simulink library "lib_Convection_LamFlatPlate"  (R2015a)
settings: Solver=ode45  StartTime=0.0  StopTime=10.0  RelTol=1e-3
libraries: simulink x1
settings Model: Creator=jlkratz  LastModifiedBy=jlkratz

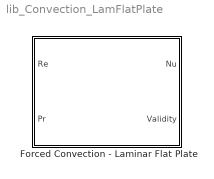
== system lib_Convection_LamFlatPlate ==
  Forced Convection - Laminar Flat Plate : Subsystem  mask(TSAT: Forced Convection - Laminar Flat Plate){LocalOrAvg_M=Average Nusselt number, IsothermOrIsoflux_M=Isothermal Plate}
      mask help:
      | This block estimates the Nusselt number of a laminar external flow over an isothermal or isoflux flat plate. It can either calculate the local or average Nusselt number over 1 surface of the plate. If the average Nusselt number is to be calcualted then assure the charateristic length used to calculate the Reynolds Number is the full length of the plate. Note that all fluid properrties should be evaluated at film temperature (average of the bulk fluid and surface temperatures). Beyond the flow being laminar the implemented correlations also requires:
      |
      | Pr >= 0.6
      |
      | If this contraint is not met then the "Validity" output will be 1, and otherwise will be 0. For more information on the implemented correlations and function of the block, see the block help menu.
      mask Help: web(which('Convection_TSAT_LaminarFlatPlate.html'),'-helpbrowser')
      mask TypeOptions LocalOrAvg_M: Local Nusselt number | Average Nusselt number
      mask TypeOptions IsothermOrIsoflux_M: Isothermal Plate | Isoflux Plate

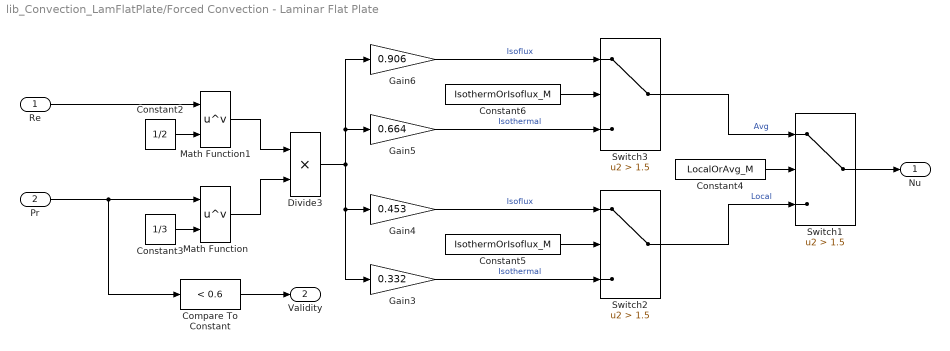
== system lib_Convection_LamFlatPlate/Forced Convection - Laminar Flat Plate ==
  Re : Inport
  Pr : Inport  Port=2
  Compare To Constant : simulink/Logic and Bit Operations/Compare To Constant  relop=<  const=0.6  OutDataTypeStr=boolean
  Constant2 : Constant  Value=1/2
  Constant3 : Constant  Value=1/3
  Constant4 : Constant  Value=LocalOrAvg_M
  Constant5 : Constant  Value=IsothermOrIsoflux_M
  Constant6 : Constant  Value=IsothermOrIsoflux_M
  Divide3 : Product  Inputs=**
  Gain3 : Gain  Gain=0.332
  Gain4 : Gain  Gain=0.453
  Gain5 : Gain  Gain=0.664
  Gain6 : Gain  Gain=0.906
  Math Function : Math  Operator=pow  SaturateOnIntegerOverflow=on
  Math Function1 : Math  Operator=pow  SaturateOnIntegerOverflow=on
  Switch1 : Switch  Criteria=u2 > Threshold  Threshold=1.5
  Switch2 : Switch  Criteria=u2 > Threshold  Threshold=1.5
  Switch3 : Switch  Criteria=u2 > Threshold  Threshold=1.5
  Nu : Outport
  Validity : Outport  Port=2
  wires:
  Gain6/1 -> Switch3/1  "Isoflux"
  Gain5/1 -> Switch3/3  "Isothermal"
  Constant6/1 -> Switch3/2
  Gain3/1 -> Switch2/3  "Isothermal"
  Gain4/1 -> Switch2/1  "Isoflux"
  Constant5/1 -> Switch2/2
  Switch2/1 -> Switch1/3  "Local"
  Switch3/1 -> Switch1/1  "Avg"
  Constant4/1 -> Switch1/2
  Divide3/1 -> Gain5/1, Gain6/1, Gain3/1, Gain4/1
  Math Function/1 -> Divide3/2
  Math Function1/1 -> Divide3/1
  Constant2/1 -> Math Function1/2
  Switch1/1 -> Nu/1
  Constant3/1 -> Math Function/2
  Pr/1 -> Compare To Constant/1, Math Function/1
  Re/1 -> Math Function1/1
  Compare To Constant/1 -> Validity/1
